simulink library "tqd"  (R2021b)
settings: Solver=VariableStepAuto  StartTime=0.0  StopTime=10.0  RelTol=1e-3
undefined symbols (not defined in the file or in its folder): ATQD_APSDecReq_X_kph, ATQD_APSDecReq_Y_mps2, ATQD_APSDecReqCMD_X_kph, ATQD_APSDecReqTs_X_pct, ATQD_APSDecTimeGain_X_Deg, ATQD_APSDecTimeGain_Y_s, ATQD_APSReqLowSpd_X_Deg, ATQD_AutoHoldReleaseBPS_X_Deg, ATQD_AWDLoadTrqnsGain_X_kg, ATQD_AWDLoadTrqnsGain_Y_pct, ATQD_BOSEnBPSPosn_X_kph, ATQD_BOSMap_X_rpm, ATQD_BOSMap_Y_pct, ATQD_CreepBaseTqD_X_kph, ATQD_CreepBaseTqD_Y_Deg, ATQD_CreepBaseTqR_X_kph, ATQD_CreepBaseTqR_Y_Deg, ATQD_CreepBPSDisPosn_X_Deg, ATQD_CreepBPSDisPosnR_X_Deg, ATQD_CreepBPSEnPosn_X_Deg, ATQD_CreepBPSEnPosnR_X_Deg, ATQD_CreepDeltaTq_X_kph, ATQD_CreepIterm_X_kph, ATQD_CreepIterm_Y_kph, ATQD_CreepItermMaxLimit_X_pct, ATQD_CreepPreloadTime_X_kph, ATQD_CreepPreloadTq_X_kph, ATQD_CreepPreloadTq_Y_s, ATQD_CreepProtTq_X_Deg, ATQD_CreepPterm_X_kph, ATQD_CreepPterm_Y_kph, ATQD_ECOTqMapD_X_rpm, ATQD_ECOTqMapD_Y_pct, ATQD_EOPDTqMapDCon_X_rpm, ATQD_EOPDTqMapDCon_Y_Deg, ATQD_EstInitVehWeight_X_c, ATQD_LHMRollGenMapD_X_rpm, ATQD_LHMRollGenMapD_Y_rpm, ATQD_LHMTqMapD_X_rpm, ATQD_LHMTqMapD_Y_pct, ATQD_NL1TqMapD_X_rpm, ATQD_NL1TqMapD_Y_pct, ATQD_NOPDTqMapDCon_X_rpm, ATQD_NOPDTqMapDCon_Y_Deg, ATQD_NRMRrEDUSpRat_X_rpm, ATQD_NRMRrEDUSpRat_Y_Nm, ATQD_OPDHoldDownRelDelay_X_Deg, ATQD_OPDHoldEnSpd_X_Deg, ATQD_OPDHoldRelDetTime_X_Deg, ATQD_OPDHoldReleaseTq_X_Deg, ATQD_OrigPedTqLowLim_X_Deg, ATQD_OrigPedTqLowLim_Y_pct, ATQD_PedalMapClimbUpLim_X_rpm, ATQD_PedalMapClimbUpLim_Y_Deg, ATQD_PreLoadTq_X_s, ATQD_RollGenMapEL1_X_rpm, ATQD_RollGenMapEL1_Y_rpm, ATQD_SL1TqMapD_X_rpm, ATQD_SL1TqMapD_Y_pct, ATQD_SlideRegenTqGain_X_Gps ... (+491)
libraries: hcu_lib x83, simulink x73, tqr x1
(part 16 of 19)

== stateflow chart tqd/TQD/TorqueDemand/Signal_convert/SWC_Subsystem/Speed Setting Mode/CC Speed Setting ON/CC Speed Setting Mode ==
  state CC
    en:
    VTQD_CCSetSpd_kph = 0;
    VTQD_CCSavedSetSpd_kph = 0;
    VTQD_CCSpdResetFinish_flg = 0;
    state Active
      (default) -> (junction 61)
      (junction 61) -> (junction 65) [order 1] : [VTQD_SWCResUpPress_enum == ENUM_SWCBOTTONPRESS_LONGPRESS  ||...
          |  VTQD_SWCResUpPress_enum == ENUM_SWCBOTTONPRESS_SHORTPRESS ||...
          | VTQD_SWCSetDownPress_enum == ENUM_SWCBOTTONPRESS_LONGPRESS  ||...
          |  VTQD_SWCSetDownPress_enum == ENUM_SWCBOTTONPRESS_SHORTPRESS   ]
      (junction 65) -> (junction 69) [order 1] : [VTQD_SWCSetDownPress_enum == ENUM_SWCBOTTONPRESS_LONGPRESS  ||...
          |  VTQD_SWCSetDownPress_enum == ENUM_SWCBOTTONPRESS_SHORTPRESS ]
      (junction 61) -> (junction 63) [order 2]
      (junction 65) -> (junction 67) [order 2]
      (junction 69) -> (junction 80)
      (junction 67) -> (junction 71) [order 1] : [VTQD_SWCResUpPress_enum == ENUM_SWCBOTTONPRESS_LONGPRESS]
      (junction 80) -> (junction 82) [order 1] : [VTQD_SWCSetDownPress_enum == ENUM_SWCBOTTONPRESS_LONGPRESS]
      (junction 67) -> (junction 73) [order 2] : %ADD_Short
          | {VTQD_CCSetSpd_kph = VTQD_CCSetSpd_kph + KTQD_SetSpdDeltaShort_kph; ...
          | VTQD_CCSetSpd_kph = min (KTQD_CCActiveMetSpdHi_raw32,VTQD_CCSetSpd_kph);...
          | VTQD_CCSavedSetSpd_kph = VTQD_CCSetSpd_kph;
          | VTQD_DistanceUnit_flg = VINP_Distanceunit_flg
          | }
      (junction 80) -> (junction 83) [order 2] : %SUBSTRACT_Short
          | {VTQD_CCSetSpd_kph = VTQD_CCSetSpd_kph - KTQD_SetSpdDeltaShort_kph; ...
          | VTQD_CCSetSpd_kph = max (KTQD_CCActiveMetSpdLo_raw32,VTQD_CCSetSpd_kph);...
          | VTQD_CCSavedSetSpd_kph = VTQD_CCSetSpd_kph;
          | VTQD_DistanceUnit_flg = VINP_Distanceunit_flg
          | }
      (junction 71) -> (junction 272)
      (junction 82) -> (junction 278)
      (junction 272) -> (junction 274) [order 1] : [VTQD_SetSpdDeltaLongFit_kph != 0]
      (junction 278) -> (junction 282) [order 1] : [VTQD_SetSpdDeltaLongFit_kph != 0]
      (junction 272) -> (junction 75) [order 2] : %ADD_Long
          | {VTQD_CCSetSpd_kph = VTQD_CCSetSpd_kph + KTQD_SetSpdDeltaLong_kph; ...
          | VTQD_CCSetSpd_kph = min (KTQD_CCActiveMetSpdHi_raw32,VTQD_CCSetSpd_kph);...
          | VTQD_CCSavedSetSpd_kph = VTQD_CCSetSpd_kph;
          | VTQD_DistanceUnit_flg = VINP_Distanceunit_flg
          | }
      (junction 274) -> (junction 276) : {
          | VTQD_CCSetSpd_kph = VTQD_CCSetSpd_kph + (KTQD_SetSpdDeltaLongFit_kph-VTQD_SetSpdDeltaLongFit_kph); ...
          | VTQD_CCSetSpd_kph = min (KTQD_CCActiveMetSpdHi_raw32,VTQD_CCSetSpd_kph); ...
          | VTQD_CCSavedSetSpd_kph = VTQD_CCSetSpd_kph;
          | VTQD_DistanceUnit_flg = VINP_Distanceunit_flg
          | }
          | %add20231127
      (junction 278) -> (junction 85) [order 2] : %SUBSTRACT_Long
          | {VTQD_CCSetSpd_kph = VTQD_CCSetSpd_kph - KTQD_SetSpdDeltaLong_kph; ...
          | VTQD_CCSetSpd_kph = max (KTQD_CCActiveMetSpdLo_raw32,VTQD_CCSetSpd_kph);...
          | VTQD_CCSavedSetSpd_kph = VTQD_CCSetSpd_kph;
          | VTQD_DistanceUnit_flg = VINP_Distanceunit_flg
          | }
      (junction 282) -> (junction 284) : {VTQD_CCSetSpd_kph = VTQD_CCSetSpd_kph - VTQD_SetSpdDeltaLongFit_kph; ...
          | VTQD_CCSetSpd_kph = max (KTQD_CCActiveMetSpdLo_raw32,VTQD_CCSetSpd_kph);...
          | VTQD_CCSavedSetSpd_kph = VTQD_CCSetSpd_kph;
          | VTQD_DistanceUnit_flg = VINP_Distanceunit_flg}
          | %add20231122
    state OFForDisable
      en:
      VTQD_CCSetSpd_kph = 0;
      VTQD_CCSavedSetSpd_kph=VTQD_CCSetSpd_kph;
      VTQD_DistanceUnit_flg = VINP_Distanceunit_flg
    state ChangeFrom_ACTIVE
      (default) -> (junction 238)
      (junction 238) -> (junction 239) [order 1] : [VTQD_CCSpdResetFinish_flg]
      (junction 238) -> (junction 241) [order 2] : {VTQD_CCSetSpd_kph = VTQD_CCSavedSetSpd_kph;}
          | %add20231206
      (junction 239) -> (junction 244)
      (junction 244) -> (junction 241)
      (junction 241) -> (junction 206)
      (junction 206) -> (junction 203) [order 1] : [VTQD_SWCResUpPress_enum == ENUM_SWCBOTTONPRESS_LONGPRESS  ||...
          |  VTQD_SWCResUpPress_enum == ENUM_SWCBOTTONPRESS_SHORTPRESS ||...
          | VTQD_SWCSetDownPress_enum == ENUM_SWCBOTTONPRESS_LONGPRESS  ||...
          |  VTQD_SWCSetDownPress_enum == ENUM_SWCBOTTONPRESS_SHORTPRESS   ]
      (junction 203) -> (junction 205) [order 1] : [VTQD_SWCResUpPress_enum == ENUM_SWCBOTTONPRESS_LONGPRESS  ||...
          |  VTQD_SWCResUpPress_enum == ENUM_SWCBOTTONPRESS_SHORTPRESS ]
      (junction 203) -> (junction 209) [order 2] : {VTQD_CCSetSpd_kph = VVMC_MeterIndSpeed_raw32;
          | VTQD_CCSpdResetFinish_flg = TRUE;
          | VTQD_CCSetSpd_kph = max (KTQD_CCActiveMetSpdLo_raw32,VTQD_CCSetSpd_kph);
          | VTQD_CCSavedSetSpd_kph=VTQD_CCSetSpd_kph;
          | VTQD_DistanceUnit_flg = VINP_Distanceunit_flg}
          | %add20231206
      (junction 206) -> (junction 211) [order 2]
      (junction 205) -> (junction 210) : {VTQD_CCSetSpd_kph = VTQD_CCSavedSetSpd_kph;
          | VTQD_CCSpdResetFinish_flg = TRUE;
          | VTQD_CCSavedSetSpd_kph=VTQD_CCSetSpd_kph;
          | VTQD_DistanceUnit_flg = VINP_Distanceunit_flg}
    state SetDown
    state LoopBack
    (default) -> (junction 1) : {VTQD_DistanceUnit_flg = VINP_Distanceunit_flg}
    (junction 253) -> (junction 258) [order 2]
    (junction 258) -> (junction 300)
    (junction 300) -> (junction 290) [order 1] : [VTQD_DistanceUnit_flg == VINP_Distanceunit_flg || VTQD_CCSavedSetSpd_kph <= ONE_FLOAT]
    CC -> (junction 253)
    (junction 290) -> (junction 1) : {VTQD_CCSetSpd_kph = min (KTQD_CCActiveMetSpdHi_raw32,VTQD_CCSetSpd_kph);
        | VTQD_CCSavedSetSpd_kph = VTQD_CCSetSpd_kph;}
    (junction 1) -> (junction 3) [order 1] : [VVMC_CCCtrlSta_enum != ENUM_ADASCCSTA_STANDBY &&...
        |  VVMC_CCCtrlSta_enum != ENUM_ADASCCSTA_ACTIVE &&...
        |  VVMC_CCCtrlSta_enum != ENUM_ADASCCSTA_OVRRIDE]
    (junction 300) -> (junction 289) [order 2]
    (junction 253) -> (junction 255) [order 1]
    (junction 256) -> (junction 258) : {VTQD_CCSpdResetFinish_flg = FALSE;}
    (junction 292) -> (junction 290)
    (junction 1) -> (junction 20) [order 2]
    (junction 3) -> OFForDisable
    (junction 289) -> (junction 295) [order 1] : [VINP_Distanceunit_flg == TRUE]
    (junction 289) -> (junction 340) [order 2] : {VTQD_CCSavedSetSpd_kph = (VTQD_CCSavedSetSpd_kph * MPH2KPH)}
    (junction 295) -> (junction 342) : {VTQD_CCSavedSetSpd_kph = (VTQD_CCSavedSetSpd_kph * KPH2MPH)}
    (junction 255) -> (junction 256) : [VVMC_CCCtrlSta_enum != ENUM_ADASCCSTA_STANDBY &&...
        | VTQD_CCSpdResetFinish_flg]
    (junction 20) -> (junction 228) [order 1] : [VVMC_CCCtrlSta_enum == ENUM_ADASCCSTA_ACTIVE ||...
        | VVMC_CCCtrlSta_enum == ENUM_ADASCCSTA_OVRRIDE
        | ]
    (junction 228) -> (junction 25) [order 2]
    (junction 20) -> (junction 181) [order 2]
    (junction 228) -> (junction 28) [order 1] : [VVMC_CCCtrlSta_enum == ENUM_ADASCCSTA_OVRRIDE]
    (junction 25) -> Active : {VTQD_CCSetSpd_kph = VTQD_CCSavedSetSpd_kph;
        | VTQD_CCSavedSetSpd_kph=VTQD_CCSetSpd_kph;
        | VTQD_DistanceUnit_flg = VINP_Distanceunit_flg}
    (junction 340) -> (junction 323) [order 1] : [VTQD_CCSavedSetSpd_kph < KTQD_CCActiveMetSpdLo_kph]
    (junction 342) -> (junction 311) [order 1] : [VTQD_CCSavedSetSpd_kph < KTQD_CCActiveMetSpdLoMPH_mph]
    (junction 340) -> (junction 324) [order 2]
    (junction 323) -> (junction 326) : {VTQD_CCSavedSetSpd_kph = KTQD_CCActiveMetSpdLo_kph}
    (junction 342) -> (junction 321) [order 2]
    (junction 311) -> (junction 307) : {VTQD_CCSavedSetSpd_kph = KTQD_CCActiveMetSpdLoMPH_mph}
    (junction 181) -> (junction 28) [order 1] : [VVMC_CCCtrlSta_enum == ENUM_ADASCCSTA_STANDBY]
    (junction 28) -> (junction 40) [order 1] : [VTQD_ChangeToSTANDBY_flg]
    (junction 181) -> LoopBack [order 2] : {VTQD_CCSetSpd_kph = VTQD_CCSavedSetSpd_kph;
        | VTQD_CCSavedSetSpd_kph=VTQD_CCSetSpd_kph;
        | VTQD_DistanceUnit_flg = VINP_Distanceunit_flg}
    (junction 28) -> (junction 43) [order 2]
    (junction 40) -> ChangeFrom_ACTIVE : {VTQD_CCSetSpd_kph = VTQD_CCSavedSetSpd_kph;
        | VTQD_CCSavedSetSpd_kph=VTQD_CCSetSpd_kph;
        | VTQD_DistanceUnit_flg = VINP_Distanceunit_flg}
    (junction 307) -> (junction 321)
    (junction 326) -> (junction 324)
    (junction 321) -> (junction 318)
    (junction 324) -> (junction 330)
    (junction 330) -> (junction 328) [order 1] : [VTQD_CCSavedSetSpd_kph > KTQD_CCActiveMetSpdHi_kph]
    (junction 318) -> (junction 313) [order 1] : [VTQD_CCSavedSetSpd_kph > KTQD_CCActiveMetSpdHiMPH_mph]
    (junction 330) -> (junction 334) [order 2]
    (junction 328) -> (junction 331) : {VTQD_CCSavedSetSpd_kph = KTQD_CCActiveMetSpdHi_kph}
    (junction 318) -> (junction 320) [order 2]
    (junction 313) -> (junction 316) : {VTQD_CCSavedSetSpd_kph = KTQD_CCActiveMetSpdHiMPH_mph}
    (junction 43) -> (junction 44) [order 1] : [VTQD_SWCSetDownPress_enum == ENUM_SWCBOTTONPRESS_LONGPRESS  ||...
        |  VTQD_SWCSetDownPress_enum == ENUM_SWCBOTTONPRESS_SHORTPRESS ]
    (junction 43) -> LoopBack [order 2] : {VTQD_CCSetSpd_kph = VTQD_CCSavedSetSpd_kph;
        | VTQD_CCSavedSetSpd_kph=VTQD_CCSetSpd_kph;
        | VTQD_DistanceUnit_flg = VINP_Distanceunit_flg}
    (junction 44) -> SetDown : {VTQD_CCSetSpd_kph = VVMC_MeterIndSpeed_raw32;
        | VTQD_CCSetSpd_kph = max (KTQD_CCActiveMetSpdLo_raw32,VTQD_CCSetSpd_kph);
        | VTQD_CCSavedSetSpd_kph=VTQD_CCSetSpd_kph;
        | VTQD_DistanceUnit_flg = VINP_Distanceunit_flg}
        | %add20231201
    (junction 331) -> (junction 334)
    (junction 316) -> (junction 320)
    (junction 334) -> (junction 301)
    (junction 320) -> (junction 291)
    (junction 301) -> (junction 291)
    (junction 291) -> (junction 292)
  data: KTQD_SetSpdDeltaLong_kph input; KTQD_SetSpdDeltaShort_kph input; KTQD_SetSpdDeltaLongFit_kph input; VTQD_SetSpdDeltaLongFit_kph input; VVMC_CCCtrlSta_enum input; VINP_Distanceunit_flg input; KTQD_CCActiveMetSpdHi_raw32 input; KTQD_CCActiveMetSpdLo_raw32 input; VVMC_MeterIndSpeed_raw32 input; VTQD_CCSetSpd_kph output single; VTQD_CCSavedSetSpd_kph local single; ENUM_ADASCCSTA_ACTIVE parameter; ENUM_ADASCCSTA_STANDBY parameter; VTQD_SWCSetDownPress_enum input; VTQD_SWCResUpPress_enum input; VTQD_ChangeToSTANDBY_flg input; ENUM_ADASCCSTA_OVRRIDE parameter; VTQD_CCSpdResetFinish_flg output; ENUM_SWCBOTTONPRESS_LONGPRESS parameter; ENUM_SWCBOTTONPRESS_SHORTPRESS parameter; FALSE parameter; TRUE parameter; KPH2MPH parameter; MPH2KPH parameter; VTQD_DistanceUnit_flg local boolean; ONE_FLOAT parameter; KTQD_CCActiveMetSpdHiMPH_mph parameter; KTQD_CCActiveMetSpdHi_kph parameter; KTQD_CCActiveMetSpdLoMPH_mph parameter; KTQD_CCActiveMetSpdLo_kph parameter

== stateflow chart tqd/TQD/TorqueDemand/Signal_convert/Chart ==
  state Creep_function_switch
    (default) -> (junction 12) : { VTQD_SaveCreepSW_flg =FALSE;}
    Creep_function_switch -> (junction 12)
    (junction 12) -> (junction 16) [order 1] : [VPMM_SysPowerMode_enum != ENUM_PWRSTASW_STANDBY ]
    (junction 12) -> (junction 19) [order 2] : {VTQD_CreepON_flg = TRUE;
        |  VTQD_SaveCreepSW_flg = VTQD_CreepON_flg;}
    (junction 16) -> (junction 23)
    (junction 23) -> (junction 25) [order 1] : [KTQD_CreepSW_flg_ovrdflg != TRUE]
    (junction 23) -> (junction 28) [order 2] : {VTQD_CreepON_flg = KTQD_CreepSW_flg_ovrdval;}
    (junction 25) -> (junction 30)
    (junction 30) -> (junction 32) [order 1] : [VINP_RegenMode_enum != ENUM_REGENLEVEL_OPD]
    (junction 30) -> (junction 34) [order 2] : {VTQD_CreepON_flg = FALSE;}
    (junction 32) -> (junction 37)
    (junction 37) -> (junction 39) [order 1] : [VTQD_OPDOn2Off_flg != TRUE]
    (junction 37) -> (junction 42) [order 2] : {VTQD_CreepON_flg = VTQD_SaveCreepSW_flg;}
    (junction 39) -> (junction 45)
    (junction 45) -> (junction 47) [order 1] : [VINP_IVICreepSWReq_flg == TRUE]
    (junction 45) -> (junction 49) [order 2] : {VTQD_CreepON_flg = VTQD_LastCreepON_flg;}
    (junction 47) -> (junction 51)
    (junction 51) -> (junction 53) [order 1] : [VTQD_LastCreepON_flg != FALSE]
    (junction 51) -> (junction 55) [order 2] : {VTQD_CreepON_flg = TRUE;
        |  VTQD_SaveCreepSW_flg = VTQD_CreepON_flg;}
    (junction 53) -> (junction 57) : {VTQD_CreepON_flg = FALSE;
        |  VTQD_SaveCreepSW_flg = VTQD_CreepON_flg;}
  (default) -> Creep_function_switch
  data: VPMM_SysPowerMode_enum input; KTQD_CreepSW_flg_ovrdflg input; KTQD_CreepSW_flg_ovrdval input; VTQD_OPDOn2Off_flg input; VINP_RegenMode_enum input; VTQD_LastCreepON_flg input; VINP_IVICreepSWReq_flg input; ENUM_PWRSTASW_STANDBY parameter; TRUE parameter; VTQD_CreepON_flg output boolean; ENUM_REGENLEVEL_OPD parameter; FALSE parameter; VTQD_SaveCreepSW_flg local boolean

== stateflow chart tqd/TQD/TorqueDemand/ShiftModule/Determine_Actual_Gear_Position ==
  state Initialize [commented out]
    en:
    VTQD_GearActualPosn_enum = ENUM_GEARACTUALPOSN_INVALID;
    VTQD_ShiftInitialComplete_flg = FALSE;
    (default) -> (junction 489) [commented out] : {
        | VTQD_InitializeTime_s = 0;
        | }
    Initialize -> (junction 489) [commented out]
    (junction 489) -> (junction 490) [commented out] : [VTQD_InitializeTime_s > KTQD_ShiftInitialTime_s]
    (junction 489) -> (junction 531) [commented out] : {
        | VTQD_InitializeTime_s = VTQD_InitializeTime_s + task_time_s;
        | }
    (junction 490) -> (junction 533) [commented out] : {
        | VTQD_ShiftInitialComplete_flg = TRUE;
        | }
    (junction 533) -> (junction 531) [commented out]
  state PBW_Judgement [commented out]
    en:
    VTQD_PBWReleased_flg = FALSE;
    VTQD_PBWLocked_flg = FALSE;
    VTQD_PBWUnlockTO_flg = FALSE;
    VTQD_PBWLockTO_flg = FALSE;
    state Initialize [commented out]
      en:
      VTQD_PBWUnlockTO_flg = FALSE;
      VTQD_PBWReleased_flg = FALSE;
      VTQD_PBWLocked_flg = FALSE;
    state PBWUnlock [commented out]
      en:
      VTQD_ParkRequest_flg = FALSE;
      (default) -> (junction 798) [commented out] : {
          | VTQD_PBWWaitTime_s = 0;
          | }
      PBWUnlock -> (junction 798) [commented out]
      (junction 798) -> (junction 799) [commented out] : [VINP_PBWMotorPos_enum == ENUM_PBWPOSITION_UNPARKED]
      (junction 798) -> (junction 800) [commented out] : {
          | VTQD_PBWWaitTime_s += task_time_s;
          | }
      (junction 799) -> (junction 804) [commented out] : {
          | VTQD_PBWReleased_flg = TRUE;
          | }
      (junction 800) -> (junction 801) [commented out] : [VTQD_PBWWaitTime_s >= KTQD_PBWTimeout_s]
      (junction 800) -> (junction 802) [commented out]
      (junction 801) -> (junction 803) [commented out] : {
          | VTQD_PBWUnlockTO_flg = TRUE;
          | }
      (junction 803) -> (junction 802) [commented out]
      (junction 804) -> (junction 803) [commented out]
    state PBWLock [commented out]
      en:
      VTQD_ParkRequest_flg = TRUE;
      (default) -> (junction 817) [commented out] : {
          | VTQD_PBWWaitTime_s = 0;
          | }
      (junction 817) -> (junction 816) [commented out] : [VINP_PBWMotorPos_enum == ENUM_PBWPOSITION_PARKED]
      PBWLock -> (junction 817) [commented out]
      (junction 816) -> (junction 822) [commented out] : {
          | VTQD_PBWLocked_flg = TRUE;
          | }
      (junction 817) -> (junction 818) [commented out] : {
          | VTQD_PBWWaitTime_s += task_time_s;
          | }
      (junction 818) -> (junction 819) [commented out] : [VTQD_PBWWaitTime_s >= KTQD_PBWTimeout_s]
      (junction 818) -> (junction 820) [commented out]
      (junction 819) -> (junction 821) [commented out] : {
          | VTQD_PBWLockTO_flg = TRUE;
          | }
      (junction 821) -> (junction 820) [commented out]
      (junction 822) -> (junction 821) [commented out]
    (default) -> PBW_Judgement.Initialize [commented out]
    PBW_Judgement.Initialize -> PBWUnlock [commented out] : [VTQD_GearShiftCMD_enum != ENUM_GEARSHIFTCMD_P]
    PBW_Judgement.Initialize -> PBWLock [commented out] : [VTQD_GearShiftCMD_enum == ENUM_GEARSHIFTCMD_P]
  state N
    en:
    VTQD_GearActualPosn_enum = ENUM_GEARACTUALPOSN_N;
    VTQD_ParkRequest_flg = FALSE;
    VTQD_EnterP_flg = FALSE;
    (default) -> (junction 753) : {
        | VTQD_RelockWaitTime_s = 0;
        | }
    (junction 753) -> (junction 754) [order 1] : %[!VTQD_PBWLockTO_flg]
    N -> (junction 753) [order 1]
    (junction 753) -> (junction 755) [order 2] : {
        | VTQD_RelockWaitTime_s += task_time_s;
        | }
    (junction 754) -> (junction 757) : {
        | VTQD_EnterP_flg = TRUE;
        | }
    (junction 755) -> (junction 756) [order 1] : [VTQD_RelockWaitTime_s >= KTQD_RelockWaitTime_s]
    (junction 755) -> (junction 760) [order 2]
    (junction 756) -> (junction 758) : {
        | VTQD_EnterP_flg = TRUE;
        | }
    (junction 758) -> (junction 760)
    (junction 757) -> (junction 758)
  state P
    en:
    VTQD_GearActualPosn_enum = ENUM_GEARACTUALPOSN_P;
    VTQD_ParkRequest_flg = TRUE;
    VTQD_ExitP_flg = FALSE;
    (default) -> (junction 636) : {
        | VTQD_ReunlockWaitTime_s = 0;
        | }
    P -> (junction 636) [order 1]
    (junction 636) -> (junction 641) [order 1] : %[!VTQD_PBWUnlockTO_flg]
    (junction 636) -> (junction 645) [order 2] : {
        | VTQD_ReunlockWaitTime_s += task_time_s;
        | }
    (junction 641) -> (junction 637) : {
        | VTQD_ExitP_flg = TRUE;
        | }
    (junction 645) -> (junction 632) [order 1] : [VTQD_ReunlockWaitTime_s >= KTQD_ReunlockWaitTime_s]
    (junction 645) -> (junction 647) [order 2]
    (junction 632) -> (junction 643) : {
        | VTQD_ExitP_flg = TRUE;
        | }
    (junction 643) -> (junction 647)
    (junction 637) -> (junction 643)
  state D
    en:
    VTQD_GearActualPosn_enum = ENUM_GEARACTUALPOSN_D;
    VTQD_ParkRequest_flg = FALSE;
  state R
    en:
    VTQD_GearActualPosn_enum = ENUM_GEARACTUALPOSN_R;
    VTQD_ParkRequest_flg = FALSE;
  (default) -> P : {
      |  VTQD_PBWLockTO_flg = FALSE;
      |  VTQD_PBWUnlockTO_flg = FALSE;
      | }
  N -> (junction 731) [order 2] : [VTQD_GearShiftCMD_enum == ENUM_GEARSHIFTCMD_R && VTQD_PwrStaAllowDR_flg &&...
      |  VTQD_TMRotateDirction_enum ~= ENUM_TMROTATEDIRECTACT_FORWARD &&...
      | (VTQD_BrkSwSta_flg || VVMC_APSActive_flg) && !VINP_EPBCarWashMode_flg]
  P -> N [order 1] : [(VTQD_GearShiftCMD_enum == ENUM_GEARSHIFTCMD_N &&...
      | VTQD_PwrStaAllowPN_flg && (VTQD_BrkSwSta_flg || VVMC_APSActive_flg) && VTQD_ExitP_flg)&&...
      | !VTQD_ForceP_flg]
      | %add20240308
  (junction 731) -> (junction 733)
  (junction 749) -> N
  N -> P [order 3] : [(VTQD_GearShiftCMD_enum == ENUM_GEARSHIFTCMD_P && VTQD_PwrStaAllowPN_flg &&...
      |  VINP_VehSpd_kph <= KTQD_VehSpd2P_kph && VTQD_EnterP_flg) || VTQD_ForceP_flg ]
      | %add20240308
  (junction 747) -> (junction 749)
  D -> N [order 1] : [VTQD_GearShiftCMD_enum == ENUM_GEARSHIFTCMD_N ||...
      | !VTQD_PwrStaAllowDR_flg ||...
      | VINP_EPBCarWashMode_flg]
  N -> D [order 1] : [VTQD_GearShiftCMD_enum == ENUM_GEARSHIFTCMD_D && VTQD_PwrStaAllowDR_flg &&...
      |  VTQD_TMRotateDirction_enum ~= ENUM_TMROTATEDIRECTACT_REVERSE &&...
      | !VINP_EPBCarWashMode_flg]
  P -> D [order 2] : [VTQD_GearShiftCMD_enum == ENUM_GEARSHIFTCMD_D &&...
      | VTQD_PwrStaAllowDR_flg && (VTQD_BrkSwSta_flg || VVMC_APSActive_flg) && VTQD_ExitP_flg &&...
      |  !VTQD_ForceP_flg]
      | %add20240308
  D -> P [order 2] : [(VTQD_GearShiftCMD_enum == ENUM_GEARSHIFTCMD_P && VTQD_PwrStaAllowPN_flg &&...
      |  VINP_VehSpd_kph <= KTQD_VehSpd2P_kph) || VTQD_ForceP_flg]
      | %add20240308
  R -> D [order 3] : [VTQD_GearShiftCMD_enum == ENUM_GEARSHIFTCMD_D && VTQD_PwrStaAllowDR_flg &&...
      | ( VTQD_BrkSwSta_flg ||VVMC_APSActive_flg) &&...
      | VINP_VehSpd_kph <= KTQD_VehSpdRev_kph]
  D -> R [order 3] : [VTQD_GearShiftCMD_enum == ENUM_GEARSHIFTCMD_R && VTQD_PwrStaAllowDR_flg &&...
      |  (VTQD_BrkSwSta_flg || VVMC_APSActive_flg) &&...
      | VINP_VehSpd_kph <= KTQD_VehSpdRev_kph]
  P -> R [order 3] : [VTQD_GearShiftCMD_enum == ENUM_GEARSHIFTCMD_R &&...
      | VTQD_PwrStaAllowDR_flg && (VTQD_BrkSwSta_flg || VVMC_APSActive_flg) && VTQD_ExitP_flg && !VTQD_ForceP_flg]
      | %add20240308
  R -> (junction 747) [order 1] : [VTQD_GearShiftCMD_enum == ENUM_GEARSHIFTCMD_N ||...
      | !VTQD_PwrStaAllowDR_flg ||...
      | VINP_EPBCarWashMode_flg]
  (junction 733) -> R
  R -> P [order 2] : [(VTQD_GearShiftCMD_enum == ENUM_GEARSHIFTCMD_P && VTQD_PwrStaAllowPN_flg &&...
      |  VINP_VehSpd_kph <= KTQD_VehSpd2P_kph) || VTQD_ForceP_flg]
      | %add20240308
  data: task_time_s input; VTQD_BrkSwSta_flg input; VTQD_GearShiftCMD_enum input; VINP_VehSpd_kph input; VINP_PBWMotorPos_enum input; VTQD_PwrStaAllowDR_flg input; VTQD_PwrStaAllowPN_flg input; VTQD_TMRotateDirction_enum input; VTQD_GearActualPosn_enum output uint8; ENUM_GEARACTUALPOSN_N parameter; ENUM_GEARACTUALPOSN_D parameter; ENUM_GEARACTUALPOSN_R parameter; ENUM_GEARACTUALPOSN_P parameter; KTQD_VehSpd2P_kph input; VTQD_InitializeTime_s local single; ENUM_GEARACTUALPOSN_INVALID parameter; FALSE parameter; TRUE parameter; VTQD_ShiftInitialComplete_flg local boolean; ENUM_GEARSHIFTCMD_D parameter; ENUM_GEARSHIFTCMD_P parameter; ENUM_GEARSHIFTCMD_R parameter; ENUM_GEARSHIFTCMD_N parameter; KTQD_VehSpdRev_kph input; KTQD_ShiftInitialTime_s input; ENUM_PBWPOSITION_PARKED parameter; ENUM_PBWPOSITION_UNPARKED parameter; VTQD_PBWLockTO_flg output boolean; VTQD_PBWUnlockTO_flg output boolean; KTQD_PBWTimeout_s input; KTQD_RelockWaitTime_s input; KTQD_ReunlockWaitTime_s input; VTQD_ParkRequest_flg output boolean; VTQD_EnterP_flg local boolean; VTQD_ExitP_flg local boolean; VTQD_PBWLocked_flg local boolean; VTQD_PBWReleased_flg local boolean; VTQD_PBWWaitTime_s local single; VTQD_RelockWaitTime_s local single; VTQD_ReunlockWaitTime_s local single; ENUM_TMROTATEDIRECTACT_FORWARD parameter; ENUM_TMROTATEDIRECTACT_REVERSE parameter; VINP_EPBCarWashMode_flg input; VVMC_APSActive_flg input; VTQD_ForceP_flg input

== stateflow chart tqd/TQD/TorqueDemand/Signal_convert/SWC2_Subsystem/Speed Control Mode ==
  state OFF
    en:
    VTQD_SpdCtrlMode_enum = ENUM_SPDCTRLMODE_OFF;
    VTQD_SpdCtrlSta_flg = FALSE;
  state ACC
    en:
    VTQD_SpdCtrlMode_enum = ENUM_SPDCTRLMODE_ACC;
    VTQD_SpdCtrlSta_flg = TRUE;
  state MSA
    en:
    VTQD_SpdCtrlMode_enum = ENUM_SPDCTRLMODE_MSA;
    VTQD_SpdCtrlSta_flg = TRUE;
  state ISA
    en:
    VTQD_SpdCtrlMode_enum = ENUM_SPDCTRLMODE_ISA;
    VTQD_SpdCtrlSta_flg = TRUE;
  (default) -> OFF
  (junction 117) -> OFF
  (junction 26) -> (junction 117) [order 1] : [
      |  VPMM_PowerSta_enum != ENUM_POWERSTA_READY || ...
      |  VTQD_ShiftGearPosn_enum == ENUM_GEARPOSNTOCAN_P
      | ]
  ACC -> OFF [order 2] : [
      | VPMM_PowerSta_enum != ENUM_POWERSTA_READY || ...
      | VTQD_ShiftGearPosn_enum != ENUM_GEARPOSNTOCAN_D
      | ]
  OFF -> ACC : [
      | VPMM_PowerSta_enum == ENUM_POWERSTA_READY && ...
      | VTQD_ShiftGearPosn_enum == ENUM_GEARPOSNTOCAN_D
      | ]
  (junction 26) -> ACC [order 2]
  (junction 100) -> (junction 26)
  ACC -> (junction 11) [order 1] : [VTQD_LScrollPressLong_flg && ...
      | VVMC_MSACtrlSta_enum != ENUM_ADASMSASTA_ACTIVE]
  (junction 11) -> (junction 14) [order 2]
  (junction 11) -> MSA [order 1] : [
      | (VINP_ADASISASta_enum == ENUM_ADASISASTA_DISABLE ||...
      | VINP_ADASISASta_enum == ENUM_ADASISASTA_ERROR || ...
      | !VTQD_IVIISAOffsetSpdCHOOSE_flg)
      | ]
  (junction 14) -> ISA : [
      | VINP_ADASISASta_enum == ENUM_ADASISASTA_OFF  && ...
      | VTQD_IVIISAOffsetSpdCHOOSE_flg
      | ]
  MSA -> ISA [order 2] : [
      | VINP_ADASISASta_enum == ENUM_ADASISASTA_OFF  && ...
      | VTQD_IVIISAOffsetSpdCHOOSE_flg
      | ]
  ISA -> (junction 100) [order 2] : [
      | VINP_ADASISASta_enum == ENUM_ADASISASTA_ERROR || ...
      | VINP_ADASISASta_enum == ENUM_ADASISASTA_DISABLE || ...
      | !VTQD_IVIISAOffsetSpdCHOOSE_flg
      | ]
  (junction 24) -> (junction 100)
  MSA -> (junction 19) [order 1]
  ISA -> (junction 21) [order 1]
  (junction 19) -> (junction 21)
  (junction 21) -> (junction 24) : [
      |  VPMM_PowerSta_enum != ENUM_POWERSTA_READY || ...
      |  VTQD_ShiftGearPosn_enum == ENUM_GEARPOSNTOCAN_P ||...
      |  VTQD_SWC2LADASSta_flg
      |  ]
  data: VPMM_PowerSta_enum input; VTQD_LScrollPressLong_flg input; ENUM_SPDCTRLMODE_OFF parameter; ENUM_SPDCTRLMODE_ACC parameter; ENUM_SPDCTRLMODE_ISA parameter; ENUM_SPDCTRLMODE_MSA parameter; FALSE parameter; ENUM_POWERSTA_READY parameter; VINP_ADASISASta_enum input; VTQD_SpdCtrlMode_enum output uint8; VTQD_SpdCtrlSta_flg output boolean; TRUE parameter; VTQD_IVIISAOffsetSpdCHOOSE_flg input; ENUM_ADASISASTA_ERROR parameter; ENUM_ADASISASTA_OFF parameter; VTQD_ShiftGearPosn_enum input; ENUM_GEARPOSNTOCAN_D parameter; ENUM_GEARPOSNTOCAN_P parameter; ENUM_ADASISASTA_DISABLE parameter; VTQD_SWC2LADASSta_flg input; VVMC_MSACtrlSta_enum input; ENUM_ADASMSASTA_ACTIVE parameter

== stateflow chart tqd/TQD/TorqueDemand/Signal_convert/SWC_Subsystem/Speed Setting Mode/CC Speed Setting ON/Specific_STATE_ChangeToSTANDBY ==
  state FLG_ON
    en:
    VTQD_CCChangeToSTANDBY_flg = TRUE;
  state Initialize
    en:
    VTQD_CCChangeToSTANDBY_flg = FALSE;
  state STAY
  (default) -> Initialize
  Initialize -> STAY : [VVMC_CCCtrlSta_enum == ENUM_ADASCCSTA_ACTIVE]
  STAY -> FLG_ON [order 1] : [VVMC_CCCtrlSta_enum == ENUM_ADASCCSTA_STANDBY]
  STAY -> Initialize [order 2] : [VVMC_CCCtrlSta_enum != ENUM_ADASCCSTA_ACTIVE &&...
      | VVMC_CCCtrlSta_enum != ENUM_ADASCCSTA_STANDBY ]
  (junction 11) -> Initialize
  FLG_ON -> (junction 9)
  (junction 9) -> (junction 11) : [VVMC_CCCtrlSta_enum != ENUM_ADASCCSTA_STANDBY]
  data: VVMC_CCCtrlSta_enum input; FALSE parameter; TRUE parameter; VTQD_CCChangeToSTANDBY_flg output boolean; ENUM_ADASCCSTA_ACTIVE parameter; ENUM_ADASCCSTA_STANDBY parameter
